simulink model "RLrobot"  (R2020b)
settings: Solver=ode15s  StartTime=0.0  StopTime=5  MaxStep=0.01  RelTol=1e-3  EnableMultiTasking=on
values from neighbouring files (symbols this model uses):
  Tf = 5    [ddpg_train_test.m]
  Ts = 0.2    [ddpg_train_test.m]
undefined symbols (not defined in the file or in its folder): Extr_Data_Mesh, sigbuilder_block, X, Y, Z
libraries: sm_lib x140, nesl_utility x29, simulink x13, rllib x1, walkingRobotUtils2 x1
(part 1 of 4)
settings Model: Creator=jihan  LastModifiedBy=zhug4
settings DataIOCC: LimitDataPoints=on  MaxDataPoints=10000
settings OptimizationCC: LifeSpan=inf
settings DebuggingCC: AllowSymbolicDim=off  SFUnexpectedBacktrackingDiag=warning  SFNoUnconditionalDefaultTransitionDiag=warning  SFExecutionAtInitializationDiag=none  ArithmeticOperatorsInVariantConditions=warning
settings SFSimCC: SimUseLocalCustomCode=off  CustomCodeUndefinedFunction=UseInterfaceOnly
settings RTWCC: RTWUseLocalCustomCode=off
settings CodeAppCC: StateflowObjectComments=on
settings GRTTargetCC: TargetLangStandard=C89/C90 (ANSI)
settings ConfigComp: CovMetricSettings=dw  CovSaveCumulativeToWorkspaceVar=on  CovSaveSingleToWorkspaceVar=on  CovExternalEMLEnable=off  CovSFcnEnable=off
settings SimscapeCC: SimscapeLogType=all  SimscapeLogSimulationStatistics=on  SimscapeLogDataHistory=10000

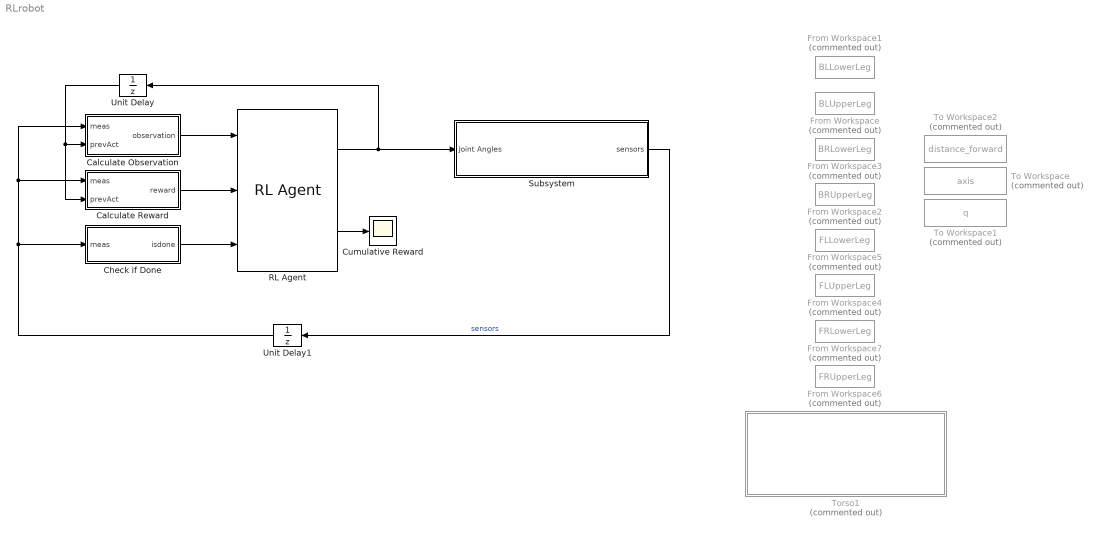
== system RLrobot ==
  Calculate Observation : Subsystem
  Calculate Reward : Subsystem
  Check if Done : Subsystem
  Cumulative Reward : Scope
  From Workspace : FromWorkspace  Commented=on  VariableName=BLUpperLeg
  From Workspace1 : FromWorkspace  Commented=on  VariableName=BLLowerLeg
  From Workspace2 : FromWorkspace  Commented=on  VariableName=BRUpperLeg
  From Workspace3 : FromWorkspace  Commented=on  VariableName=BRLowerLeg
  From Workspace4 : FromWorkspace  Commented=on  VariableName=FLUpperLeg
  From Workspace5 : FromWorkspace  Commented=on  VariableName=FLLowerLeg
  From Workspace6 : FromWorkspace  Commented=on  VariableName=FRUpperLeg
  From Workspace7 : FromWorkspace  Commented=on  VariableName=FRLowerLeg
  RL Agent : rllib/RL Agent  Agent=agent  ProvideReward=on  ProvideIsDone=on  ProvideCumRwd=on  TreatAsDirectFeedthrough=on  CollectLoggedSignals=on  CollectModelStates=on
      settings: SourceProductName=Reinforcement Learning
  Subsystem : Subsystem
  To Workspace : ToWorkspace  Commented=on  VariableName=axis  SaveFormat=Timeseries  SampleTime=1
      settings: MaxDataPoints=200
  To Workspace1 : ToWorkspace  Commented=on  VariableName=q  SaveFormat=Timeseries  SampleTime=1
      settings: MaxDataPoints=200
  To Workspace2 : ToWorkspace  Commented=on  VariableName=distance_forward  SaveFormat=Timeseries  SampleTime=1
      settings: MaxDataPoints=200
  Torso1 : Subsystem  Commented=on  mask{L=72, W=30, H=18, weight=20, rgb=[0 0.4 0.6], Lo=6, Lh=4}
      mask prompts: L "Length (cm)"; W "Width (cm)"; H "Thickness (cm)"; weight "Mass (kg)"; rgb "Color (rgb)"; Lo "Leg-Body Length offset"; Lh "Leg-Body Height offset"
      settings: PortSchema="{\"entries\":[{\"content\":{\"sides\":[{\"content\":{\"connectorIds\":[]},\"type\":\"ConnectorPlacement.EquallySpacedRectSide\",\"uuid\":\"a5f9388a-3463-4939-824e-c198da670e8b\"},{\"content\":{\"connectorIds\":[],\"side\":\"RIGHT\"},\"type\":\"ConnectorPlacement.EquallySpacedRectSide\",\"uuid\":\"721d6b97-2d6f-40dc-acf2-829076b6800c\"},{\"content\":{\"connectorIds\":[\"LConn1\",\"LConn2\"],\"side\":\"TOP\"},\"type\":\"ConnectorPlacement.EquallySpacedRectSide\",\"uuid\":\"81892bad-b270-4b55-8468-6b6312875fb4\"},{\"content\":{\"connectorIds\":[\"RConn1\",\"RConn2\",\"RConn3\",\"RConn4\"],\"side\":\"BOTTOM\"},\"type\":\"ConnectorPlacement.EquallySpacedRectSide\",\"uuid\":\"33367d70-bee6-41a0-95af-0235c6937548\"}]},\"type\":\"ConnectorPlacement.EquallySpacedConnector\",\"uuid\":\"7850cfb1-cafa-49f7-b14e-b890040a623d\"}],\"packageUris\":[\"http://schema.mathworks.com/mf0/Connector/R2020b\"],\"version\":\"1.0\"}"
  Unit Delay : UnitDelay  SampleTime=-1  HasFrameUpgradeWarning=on
  Unit Delay1 : UnitDelay  SampleTime=-1  HasFrameUpgradeWarning=on
  wires:
  Check if Done/1(isdone) -> RL Agent/3
  RL Agent/1 -> Subsystem/1(Joint Angles), Unit Delay/1
  Unit Delay/1 -> Calculate Reward/2(prevAct), Calculate Observation/2(prevAct)
  RL Agent/2 -> Cumulative Reward/1
  Calculate Observation/1(observation) -> RL Agent/1
  Calculate Reward/1(reward) -> RL Agent/2
  Subsystem/1(sensors) -> Unit Delay1/1  "sensors"
  Unit Delay1/1 -> Calculate Observation/1(meas), Calculate Reward/1(meas), Check if Done/1(meas)

== system RLrobot/Calculate Observation ==
  meas : Inport
  prevAct : Inport  Port=2
  Bus Selector : BusSelector  OutputSignals=yaw,pitch,roll,wx,wy,wz,bx,by,bz,x,y,z,vx,vy,vz,ax,ay,az
  Mux : Mux  Inputs=19
  Rate Transition : RateTransition
  Scale Height : Gain  Gain=1/0.05
  Subtract Initial Height : Bias
  observation : Outport  VectorParamsAs1DForOutWhenUnconnected=off
  wires:
  meas/1 -> Bus Selector/1
  Mux/1 -> Rate Transition/1
  Rate Transition/1 -> observation/1
  Subtract Initial Height/1 -> Scale Height/1
  prevAct/1 -> Mux/19
  Bus Selector/1 -> Mux/1  "<yaw>"
  Bus Selector/2 -> Mux/2  "<pitch>"
  Bus Selector/3 -> Mux/3  "<roll>"
  Bus Selector/4 -> Mux/4  "<wx>"
  Bus Selector/5 -> Mux/5  "<wy>"
  Bus Selector/6 -> Mux/6  "<wz>"
  Bus Selector/7 -> Mux/7  "<bx>"
  Bus Selector/8 -> Mux/8  "<by>"
  Bus Selector/9 -> Mux/9  "<bz>"
  Bus Selector/10 -> Mux/10  "<x>"
  Bus Selector/11 -> Mux/11  "<y>"
  Bus Selector/12 -> Subtract Initial Height/1  "<z>"
  Scale Height/1 -> Mux/12  "Z_scaled"
  Bus Selector/13 -> Mux/13  "<vx>"
  Bus Selector/14 -> Mux/14  "<vy>"
  Bus Selector/15 -> Mux/15  "<vz>"
  Bus Selector/16 -> Mux/16  "<ax>"
  Bus Selector/17 -> Mux/17  "<ay>"
  Bus Selector/18 -> Mux/18  "<az>"

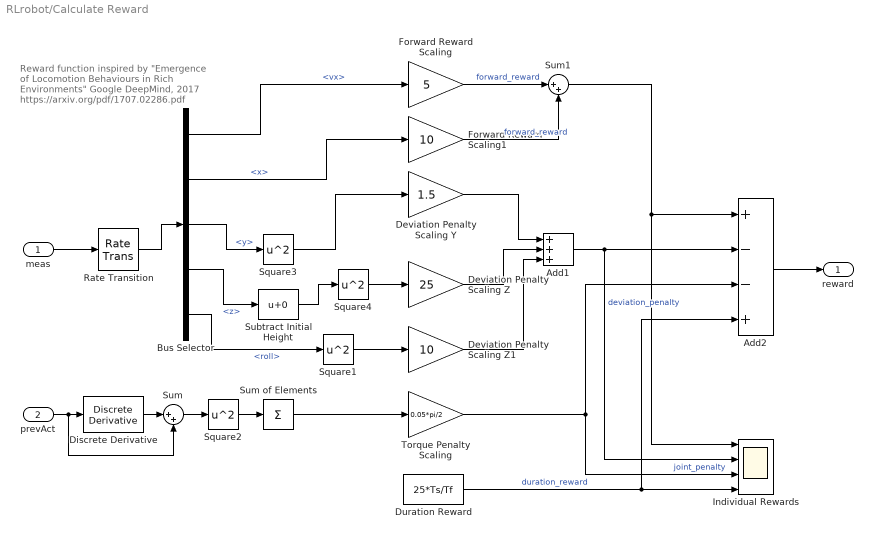
== system RLrobot/Calculate Reward ==
  note: Reward function inspired by
      | "Emergence of Locomotion Behaviours in Rich Environments"
      | Google DeepMind, 2017
      | https://arxiv.org/pdf/1707.02286.pdf
  meas : Inport
  prevAct : Inport  Port=2
  Add1 : Sum  Inputs=+++
  Add2 : Sum  Inputs=+--+
  Bus Selector : BusSelector  OutputSignals=vx,x,y,z,roll
  Deviation Penalty Scaling Y : Gain  Gain=1.5
  Deviation Penalty Scaling Z : Gain  Gain=25
  Deviation Penalty Scaling Z1 : Gain  Gain=10
  Discrete Derivative : simulink/Discrete/Discrete Derivative  gainval=1.0  ICPrevScaledInput=0.0  OutMin=[]  OutMax=[]  OutDataType=fixdt(1, 16)  OutScaling=2^-10  DoSatur=off
  Duration Reward : Constant  Value=25*Ts/Tf
  Forward Reward Scaling : Gain  Gain=5
  Forward Reward Scaling1 : Gain  Gain=10
  Individual Rewards : Scope  NumInputPorts=4
  Rate Transition : RateTransition  OutPortSampleTime=Ts
  Square{1..4} (4 alike) : Math  Operator=square  SignedPower=on  SaturateOnIntegerOverflow=on
  Subtract Initial Height : Bias
  Sum : Sum  Inputs=|++
  Sum of Elements : Sum  Inputs=+
  Sum1 : Sum  Inputs=|++
  Torque Penalty Scaling : Gain  Gain=0.05*pi/2
  reward : Outport  VectorParamsAs1DForOutWhenUnconnected=off
  wires:
  Add2/1 -> reward/1
  Add1/1 -> Add2/2, Individual Rewards/2  "deviation_penalty"
  Sum of Elements/1 -> Torque Penalty Scaling/1
  Bus Selector/1 -> Forward Reward Scaling/1  "<vx>"
  Square3/1 -> Deviation Penalty Scaling Y/1
  Duration Reward/1 -> Individual Rewards/4, Add2/4  "duration_reward"
  Square2/1 -> Sum of Elements/1
  Torque Penalty Scaling/1 -> Add2/3, Individual Rewards/3  "joint_penalty"
  Square4/1 -> Deviation Penalty Scaling Z/1
  Subtract Initial Height/1 -> Square4/1
  Deviation Penalty Scaling Z/1 -> Add1/2
  Deviation Penalty Scaling Y/1 -> Add1/1
  Bus Selector/3 -> Square3/1  "<y>"
  Bus Selector/4 -> Subtract Initial Height/1  "<z>"
  Rate Transition/1 -> Bus Selector/1
  meas/1 -> Rate Transition/1
  prevAct/1 -> Sum/2, Discrete Derivative/1
  Discrete Derivative/1 -> Sum/1
  Sum/1 -> Square2/1
  Bus Selector/2 -> Forward Reward Scaling1/1  "<x>"
  Sum1/1 -> Add2/1, Individual Rewards/1
  Forward Reward Scaling/1 -> Sum1/1  "forward_reward"
  Forward Reward Scaling1/1 -> Sum1/2  "forward_reward"
  Deviation Penalty Scaling Z1/1 -> Add1/3
  Bus Selector/5 -> Square1/1  "<roll>"
  Square1/1 -> Deviation Penalty Scaling Z1/1

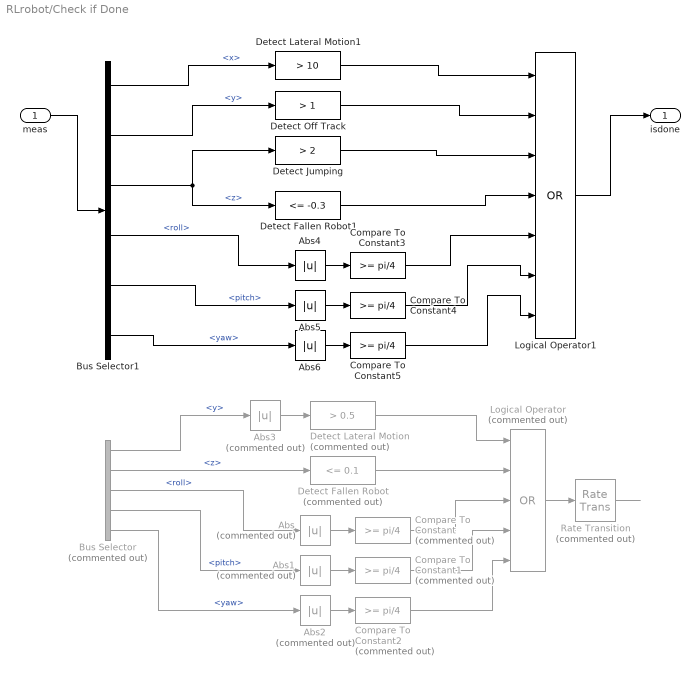
== system RLrobot/Check if Done ==
  meas : Inport
  Abs{,1..3} (4 alike) : Abs  Commented=on
  Abs4 : Abs
  Abs5 : Abs
  Abs6 : Abs
  Bus Selector : BusSelector  Commented=on  OutputSignals=y,z,roll,pitch,yaw
  Bus Selector1 : BusSelector  OutputSignals=x,y,z,roll,pitch,yaw
  Compare To Constant : simulink/Logic and Bit Operations/Compare To Constant  Commented=on  relop=>=  const=pi/4  OutDataTypeStr=boolean
  Compare To Constant1 : simulink/Logic and Bit Operations/Compare To Constant  Commented=on  relop=>=  const=pi/4  OutDataTypeStr=boolean
  Compare To Constant2 : simulink/Logic and Bit Operations/Compare To Constant  Commented=on  relop=>=  const=pi/4  OutDataTypeStr=boolean
  Compare To Constant3 : simulink/Logic and Bit Operations/Compare To Constant  relop=>=  const=pi/4  OutDataTypeStr=boolean
  Compare To Constant4 : simulink/Logic and Bit Operations/Compare To Constant  relop=>=  const=pi/4  OutDataTypeStr=boolean
  Compare To Constant5 : simulink/Logic and Bit Operations/Compare To Constant  relop=>=  const=pi/4  OutDataTypeStr=boolean
  Detect Fallen Robot : simulink/Logic and Bit Operations/Compare To Constant  Commented=on  relop=<=  const=0.1  OutDataTypeStr=boolean
  Detect Fallen Robot1 : simulink/Logic and Bit Operations/Compare To Constant  relop=<=  const=-0.3  OutDataTypeStr=boolean
  Detect Jumping : simulink/Logic and Bit Operations/Compare To Constant  relop=>  const=2  OutDataTypeStr=boolean
  Detect Lateral Motion : simulink/Logic and Bit Operations/Compare To Constant  Commented=on  relop=>  const=0.5  OutDataTypeStr=boolean
  Detect Lateral Motion1 : simulink/Logic and Bit Operations/Compare To Constant  relop=>  const=10  OutDataTypeStr=boolean
  Detect Off Track : simulink/Logic and Bit Operations/Compare To Constant  relop=>  const=1  OutDataTypeStr=boolean
  Logical Operator : Logic  Commented=on  Operator=OR  Inputs=5  AllPortsSameDT=off  OutDataTypeStr=boolean
  Logical Operator1 : Logic  Operator=OR  Inputs=7  AllPortsSameDT=off  OutDataTypeStr=boolean
  Rate Transition : RateTransition  Commented=on
  isdone : Outport  VectorParamsAs1DForOutWhenUnconnected=off
  wires:
  Bus Selector/5 -> Abs2/1  "<yaw>"
  Abs2/1 -> Compare To Constant2/1
  Abs3/1 -> Detect Lateral Motion/1
  Detect Lateral Motion/1 -> Logical Operator/1
  Bus Selector/3 -> Abs/1  "<roll>"
  Abs1/1 -> Compare To Constant1/1
  Abs/1 -> Compare To Constant/1
  Compare To Constant2/1 -> Logical Operator/5
  Logical Operator/1 -> Rate Transition/1
  Compare To Constant/1 -> Logical Operator/3
  Compare To Constant1/1 -> Logical Operator/4
  Bus Selector/1 -> Abs3/1  "<y>"
  Bus Selector/4 -> Abs1/1  "<pitch>"
  Detect Fallen Robot/1 -> Logical Operator/2
  Bus Selector/2 -> Detect Fallen Robot/1  "<z>"
  Rate Transition/1 -> ?
  meas/1 -> Bus Selector1/1
  Bus Selector1/1 -> Detect Lateral Motion1/1  "<x>"
  Detect Lateral Motion1/1 -> Logical Operator1/1
  Logical Operator1/1 -> isdone/1
  Detect Fallen Robot1/1 -> Logical Operator1/4
  Bus Selector1/2 -> Detect Off Track/1  "<y>"
  Detect Off Track/1 -> Logical Operator1/2
  Detect Jumping/1 -> Logical Operator1/3
  Bus Selector1/3 -> Detect Fallen Robot1/1, Detect Jumping/1  "<z>"
  Abs4/1 -> Compare To Constant3/1
  Compare To Constant5/1 -> Logical Operator1/7
  Compare To Constant4/1 -> Logical Operator1/6
  Abs6/1 -> Compare To Constant5/1
  Abs5/1 -> Compare To Constant4/1
  Bus Selector1/4 -> Abs4/1  "<roll>"
  Bus Selector1/5 -> Abs5/1  "<pitch>"
  Compare To Constant3/1 -> Logical Operator1/5
  Bus Selector1/6 -> Abs6/1  "<yaw>"

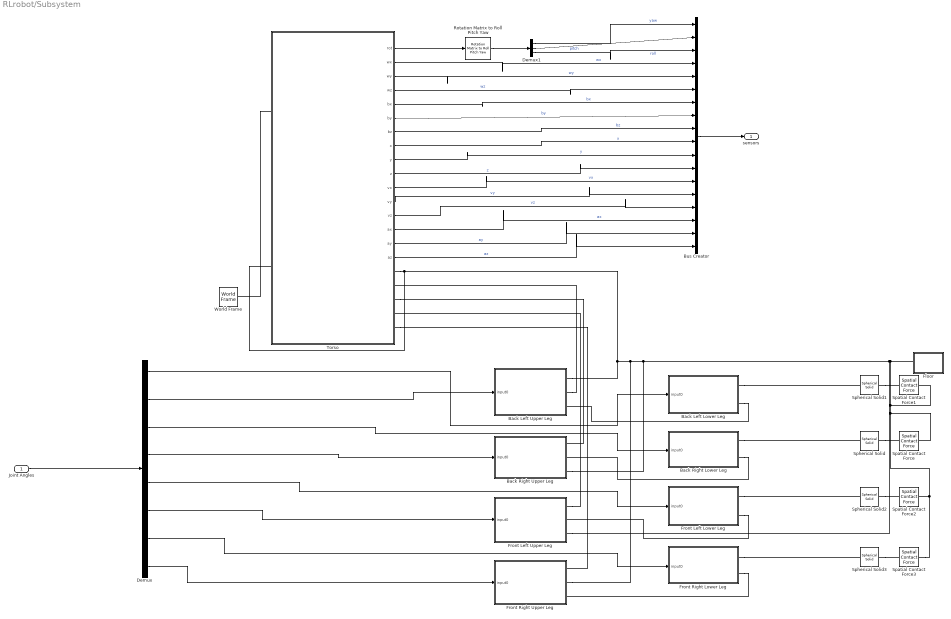
== system RLrobot/Subsystem ==
  Joint Angles : Inport  Unit=m^2*kg/s^2
  " Front Right Upper Leg" : Subsystem  mask{L=7, W=5, H=25, weight=1, rgb=[0 0.4 0.6]}
      mask prompts: L "Length (cm)"; W "Width (cm)"; H "Height (cm)"; weight "Weight (kg)"; rgb "Color (rgb)"
  Back Left Lower Leg : Subsystem  mask{L=7, W=5, H=25, weight=1, rgb=[0 0.4 0.6]}
      mask prompts: L "Length (cm)"; W "Width (cm)"; H "Height (cm)"; weight "Weight (cm)"; rgb "Color (rgb)"
  Back Left Upper Leg : Subsystem  mask{L=7, W=5, H=25, weight=1, rgb=[0 0.4 0.6]}
      mask prompts: L "Length (cm)"; W "Width (cm)"; H "Height (cm)"; weight "Weight (cm)"; rgb "Color (rgb)"
  Back Right Lower Leg : Subsystem  mask{L=7, W=5, H=25, weight=1, rgb=[0 0.4 0.6]}
      mask prompts: L "Length (cm)"; W "Width (cm)"; H "Height (cm)"; weight "Weight (cm)"; rgb "Color (rgb)"
  Back Right Upper Leg : Subsystem  mask{L=7, W=5, H=25, weight=1, rgb=[0 0.4 0.6]}
      mask prompts: L "Length (cm)"; W "Width (cm)"; H "Height (cm)"; weight "Weight (kg)"; rgb "Color (rgb)"
  Bus Creator : BusCreator  Inputs=18
  Demux : Demux  Outputs=8
  Demux1 : Demux  Outputs=3
  Floor : Subsystem  mask{xyz=[0 1 0], floor_angle=0, offset=90}
      mask prompts: xyz "Axis of Rotation [x y z]"; floor_angle "Angle of Rotation (deg)"; offset "Floor Offset (cm)"
      settings: PortSchema="{\"entries\":[{\"content\":{\"sides\":[{\"content\":{\"connectorIds\":[]},\"type\":\"ConnectorPlacement.EquallySpacedRectSide\",\"uuid\":\"11e96fa0-1698-473b-91b9-c65afd80511d\"},{\"content\":{\"connectorIds\":[],\"side\":\"RIGHT\"},\"type\":\"ConnectorPlacement.EquallySpacedRectSide\",\"uuid\":\"698adcb8-63bc-493a-8506-9415d482b8fe\"},{\"content\":{\"connectorIds\":[\"LConn1\"],\"side\":\"TOP\"},\"type\":\"ConnectorPlacement.EquallySpacedRectSide\",\"uuid\":\"168764b1-d6dd-4696-94dd-d7ccb4fea120\"}]},\"type\":\"ConnectorPlacement.EquallySpacedConnector\",\"uuid\":\"ee92c37f-2eb0-4cad-ab84-9513ea85ac02\"}],\"packageUris\":[\"http://schema.mathworks.com/mf0/Connector/19700101\"],\"version\":\"1.0\"}"
  Front Left Lower Leg : Subsystem  mask{L=7, W=5, H=25, weight=1, rgb=[0 0.4 0.6]}
      mask prompts: L "Length (cm)"; W "Width (cm)"; H "Height (cm)"; weight "Weight (kg)"; rgb "Color (rgb)"
  Front Left Upper Leg : Subsystem  mask{L=7, W=5, H=25, weight=1, rgb=[0 0.4 0.6]}
      mask prompts: L "Length (cm)"; W "Width (cm)"; H "Height (cm)"; weight "Weight (kg)"; rgb "Color (rgb)"
  Front Right Lower Leg : Subsystem  mask{L=7, W=5, H=25, weight=1, rgb=[0 0.4 0.6]}
      mask prompts: L "Length (cm)"; W "Width (cm)"; H "Height (cm)"; weight "Weight (cm)"; rgb "Color (rgb)"
  Rotation Matrix to Roll Pitch Yaw : walkingRobotUtils2/Rotation Matrix to  Roll Pitch Yaw  SystemSampleTime=-1  VariantActivationTime=update diagram  Latency=0  AutoFrameSizeCalculation=off
  Spatial Contact Force{,1..3} (4 alike) : sm_lib/Forces and Torques/Spatial Contact Force  CoefficientOfDynamicFriction=0.3  CoefficientOfStaticFriction=0.3  NormalDamping=1e3  NormalDampingUnits=N/(m/s)  NormalStiffness=1e6  NormalStiffnessUnits=N/m  FrictionalCriticalVelocity=1e-3  FrictionalCriticalVelocityUnits=m/s  ZeroCrossDetectContactStartAndEnd=off  SenseFrictionalForceMagnitude=off  SenseNormalForceMagnitude=off  SenseSeparationDistance=off  NormalTransitionRegionWidth=1e-4  NormalTransitionRegionWidthUnits=m  FrictionType=SmoothStickSlip
  Spherical Solid{,1..3} (4 alike) : sm_lib/Body Elements/Spherical Solid  GraphicAmbientColor=[0.15 0.15 0.15 1.0]  BasedOnType=Density  CenterOfMass=[0 0 0]  CenterOfMassUnits=m  GraphicDiffuseColor=[0.5 0.5 0.5]  Density=1000  DensityUnits=kg/m^3  DoExposeReferenceFrame=on  GraphicEmissiveColor=[0.0 0.0 0.0 1.0]  ExportEntireGeometry=on  SerializedExposedGeometries=<ExposedGeometries><ExposedGeometry><RawGeometryId>entire</RawGeometryId><ExposedGeometryId>G</ExposedGeometryId></ExposedGeometry></ExposedGeometries>  SerializedFrames=<Frames/>  MarkerShape=Sphere  MarkerSize=10  GraphicType=FromGeometry  InertiaType=CalculateFromGeometry  Mass=1  MassUnits=kg  MomentsOfInertia=[1 1 1]  MomentsOfInertiaUnits=kg*m^2  GraphicOpacity=1.0  ProductsOfInertia=[0 0 0]  ProductsOfInertiaUnits=kg*m^2  GraphicShininess=75  GraphicSpecularColor=[0.5 0.5 0.5 1.0]  SphereRadius=4  SphereRadiusUnits=cm  GraphicVisPropType=SimpleVisualProperties
  Torso : Subsystem  mask{L=72, W=30, H=18, weight=20, rgb=[0 0.4 0.6], Lo=6, Lh=4}
      mask prompts: L "Length (cm)"; W "Width (cm)"; H "Thickness (cm)"; weight "Mass (kg)"; rgb "Color (rgb)"; Lo "Leg-Body Length offset"; Lh "Leg-Body Height offset"
  World Frame : sm_lib/Frames and Transforms/World Frame
  sensors : Outport
  wires:
  Demux/1 -> Back Left Lower Leg/1(input0)
  Demux/3 -> Back Right Lower Leg/1(input0)
  Demux/5 -> Front Left Lower Leg/1(input0)
  Demux/4 -> Back Right Upper Leg/1(input0)
  Demux/8 -> " Front Right Upper Leg"/1(input0)
  Demux/6 -> Front Left Upper Leg/1(input0)
  Demux/7 -> Front Right Lower Leg/1(input0)
  Demux/2 -> Back Left Upper Leg/1(input0)
  Joint Angles/1 -> Demux/1
  Bus Creator/1 -> sensors/1
  Demux1/3 -> Bus Creator/3  "roll"
  Demux1/1 -> Bus Creator/1  "yaw"
  Demux1/2 -> Bus Creator/2  "pitch"
  Torso/2(wx) -> Bus Creator/4  "wx"
  Torso/3(wy) -> Bus Creator/5  "wy"
  Torso/4(wz) -> Bus Creator/6  "wz"
  Torso/5(bx) -> Bus Creator/7  "bx"
  Torso/6(by) -> Bus Creator/8  "by"
  Torso/7(bz) -> Bus Creator/9  "bz"
  Torso/8(x) -> Bus Creator/10  "x"
  Torso/9(y) -> Bus Creator/11  "y"
  Torso/10(z) -> Bus Creator/12  "z"
  Torso/11(vx) -> Bus Creator/13  "vx"
  Torso/12(vy) -> Bus Creator/14  "vy"
  Torso/13(vz) -> Bus Creator/15  "vz"
  Torso/15(ay) -> Bus Creator/17  "ay"
  Torso/14(ax) -> Bus Creator/16  "ax"
  Torso/16(az) -> Bus Creator/18  "az"
  Torso/1(rot) -> Rotation Matrix to Roll Pitch Yaw/1
  Rotation Matrix to Roll Pitch Yaw/1 -> Demux1/1
  connections:
  Back Left Lower Leg/RConn2 -- Back Left Upper Leg/RConn3
  Spatial Contact Force1/RConn1 -- Spatial Contact Force3/RConn1 -- Spatial Contact Force2/RConn1 -- Spatial Contact Force/RConn1 -- Floor/LConn1 -- Torso/RConn1 -- Torso/LConn2 -- Back Left Upper Leg/RConn1 -- " Front Right Upper Leg"/RConn2 -- Back Right Upper Leg/RConn3 -- Front Left Upper Leg/RConn3
  Spherical Solid3/LConn1 -- Spatial Contact Force3/LConn1
  Spherical Solid/LConn1 -- Spatial Contact Force/LConn1
  Back Right Lower Leg/RConn1 -- Spherical Solid/RConn1
  Spherical Solid1/LConn1 -- Spatial Contact Force1/LConn1
  Front Left Lower Leg/RConn1 -- Spherical Solid2/RConn1
  Back Left Upper Leg/RConn2 -- Torso/RConn2
  Spherical Solid2/LConn1 -- Spatial Contact Force2/LConn1
  Front Right Lower Leg/RConn2 -- " Front Right Upper Leg"/RConn3
  Back Right Lower Leg/RConn2 -- Back Right Upper Leg/RConn2
  Back Left Lower Leg/RConn1 -- Spherical Solid1/RConn1
  Front Right Lower Leg/RConn1 -- Spherical Solid3/RConn1
  Torso/RConn5 -- " Front Right Upper Leg"/RConn1
  Front Left Lower Leg/RConn2 -- Front Left Upper Leg/RConn2
  Torso/LConn1 -- World Frame/RConn1
  Front Left Upper Leg/RConn1 -- Torso/RConn4
  Torso/RConn3 -- Back Right Upper Leg/RConn1

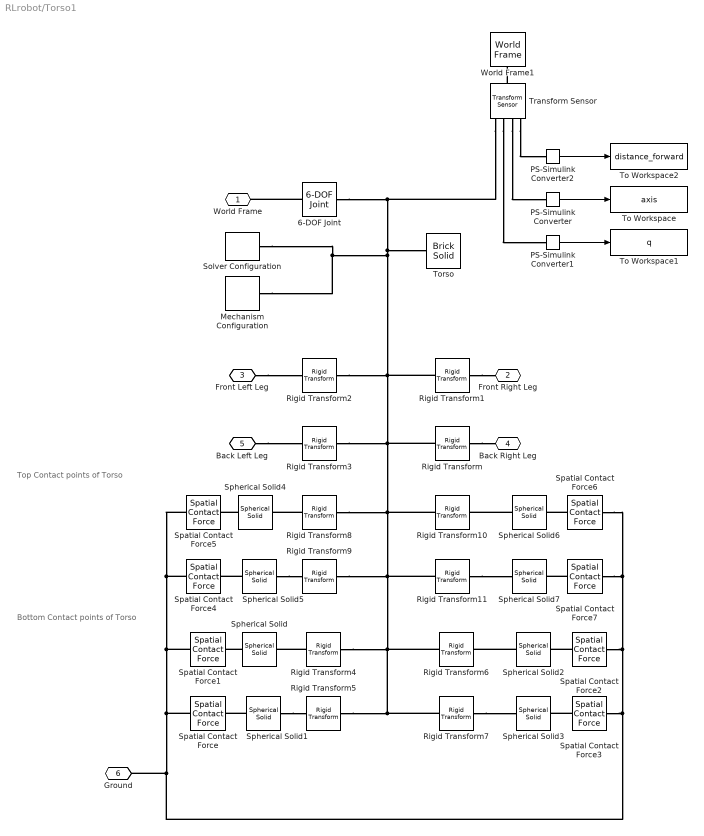
== system RLrobot/Torso1 ==
  note: Top Contact points of Torso
  note: Bottom Contact points of Torso
  6-DOF Joint : sm_lib/Joints/6-DOF Joint  JointMode=Normal  SenseConstraintForce=off  SenseConstraintForceX=off  SenseConstraintForceY=off  SenseConstraintForceZ=off  SenseConstraintTorque=off  SenseConstraintTorqueX=off  SenseConstraintTorqueY=off  SenseConstraintTorqueZ=off  SenseTotalForce=off  SenseTotalForceX=off  SenseTotalForceY=off  SenseTotalForceZ=off  SenseTotalTorque=off  SenseTotalTorqueX=off  SenseTotalTorqueY=off  SenseTotalTorqueZ=off  CompositeWrenchDir=FollowerOnBase  CompositeWrenchFrame=BaseFrame  PxEquilibriumPosition=0  PxEquilibriumPositionUnits=m  PxSpringStiffness=0  PxSpringStiffnessUnits=N/m  PxDampingCoefficient=0  PxDampingCoefficientUnits=N/(m/s)  PxTorqueActuationMode=NoTorque  PxMotionActuationMode=ComputedMotion  PxSensePosition=off  PxSenseVelocity=off  PxSenseAcceleration=off  PxSenseTorqueForce=off  PxSenseLowerLimitTorqueForce=off  PxSenseUpperLimitTorqueForce=off  PxLowerLimitSpecify=off  PxLowerLimitBound=-1  PxLowerLimitBoundUnits=m  PxLowerLimitStiffness=1e6  PxLowerLimitStiffnessUnits=N/m  PxLowerLimitDamping=1e3  PxLowerLimitDampingUnits=N/(m/s)  PxLowerLimitTransitionRegionWidth=1e-4  PxLowerLimitTransitionRegionWidthUnits=m  PxUpperLimitSpecify=off  PxUpperLimitBound=1  PxUpperLimitBoundUnits=m  PxUpperLimitStiffness=1e6  PxUpperLimitStiffnessUnits=N/m  PxUpperLimitDamping=1e3  PxUpperLimitDampingUnits=N/(m/s)  PxUpperLimitTransitionRegionWidth=1e-4  PxUpperLimitTransitionRegionWidthUnits=m  PxPositionTargetSpecify=off  PxPositionTargetPriority=High  PxPositionTargetValue=0  PxPositionTargetValueUnits=m  PxVelocityTargetSpecify=off  PxVelocityTargetPriority=High  PxVelocityTargetValue=0  PxVelocityTargetValueUnits=m/s  PyEquilibriumPosition=0  PyEquilibriumPositionUnits=m  PySpringStiffness=0  PySpringStiffnessUnits=N/m  PyDampingCoefficient=0  PyDampingCoefficientUnits=N/(m/s)  PyTorqueActuationMode=NoTorque  PyMotionActuationMode=ComputedMotion  PySensePosition=off  PySenseVelocity=off  PySenseAcceleration=off  PySenseTorqueForce=off  PySenseLowerLimitTorqueForce=off  PySenseUpperLimitTorqueForce=off  PyLowerLimitSpecify=off  PyLowerLimitBound=-1  PyLowerLimitBoundUnits=m  PyLowerLimitStiffness=1e6  PyLowerLimitStiffnessUnits=N/m  PyLowerLimitDamping=1e3  PyLowerLimitDampingUnits=N/(m/s)  PyLowerLimitTransitionRegionWidth=1e-4  PyLowerLimitTransitionRegionWidthUnits=m  PyUpperLimitSpecify=off  PyUpperLimitBound=1  PyUpperLimitBoundUnits=m  PyUpperLimitStiffness=1e6  PyUpperLimitStiffnessUnits=N/m  PyUpperLimitDamping=1e3  PyUpperLimitDampingUnits=N/(m/s)  PyUpperLimitTransitionRegionWidth=1e-4  PyUpperLimitTransitionRegionWidthUnits=m  PyPositionTargetSpecify=off  PyPositionTargetPriority=High  PyPositionTargetValue=0  PyPositionTargetValueUnits=m  PyVelocityTargetSpecify=off  PyVelocityTargetPriority=High  PyVelocityTargetValue=0  PyVelocityTargetValueUnits=m/s  PzEquilibriumPosition=0  PzEquilibriumPositionUnits=m  PzSpringStiffness=0  PzSpringStiffnessUnits=N/m  PzDampingCoefficient=0  PzDampingCoefficientUnits=N/(m/s)  PzTorqueActuationMode=NoTorque  PzMotionActuationMode=ComputedMotion  PzSensePosition=off  PzSenseVelocity=off  PzSenseAcceleration=off  PzSenseTorqueForce=off  PzSenseLowerLimitTorqueForce=off  PzSenseUpperLimitTorqueForce=off  PzLowerLimitSpecify=off  PzLowerLimitBound=-1  PzLowerLimitBoundUnits=m  PzLowerLimitStiffness=1e6  PzLowerLimitStiffnessUnits=N/m  PzLowerLimitDamping=1e3  PzLowerLimitDampingUnits=N/(m/s)  PzLowerLimitTransitionRegionWidth=1e-4  PzLowerLimitTransitionRegionWidthUnits=m  PzUpperLimitSpecify=off  PzUpperLimitBound=1  PzUpperLimitBoundUnits=m  PzUpperLimitStiffness=1e6  PzUpperLimitStiffnessUnits=N/m  PzUpperLimitDamping=1e3  PzUpperLimitDampingUnits=N/(m/s)  PzUpperLimitTransitionRegionWidth=1e-4  PzUpperLimitTransitionRegionWidthUnits=m  PzPositionTargetSpecify=off  PzPositionTargetPriority=High  PzPositionTargetValue=0  PzPositionTargetValueUnits=m  PzVelocityTargetSpecify=off  PzVelocityTargetPriority=High  PzVelocityTargetValue=0  PzVelocityTargetValueUnits=m/s  SphDefPosRotationMethod=None  SphDefPosRotationAngleUnits=deg  SphDefPosRotationStandardAxis=+Z  SphDefPosRotationAngle=0.0  SphDefPosRotationArbitraryAxis=[0 0 1]  SphDefPosFollAlignAxisA=+X  SphDefPosBaseAlignAxisA=+Y  SphDefPosFollAlignAxisB=+Y  SphDefPosBaseAlignAxisB=+Z  SphDefPosRotationSequenceAxes=FollowerAxes  SphDefPosRotationSequence=XYX  SphDefPosRotationSequenceAngles=[0 0 0]  SphDefPosRotationSequenceAnglesUnits=deg  SphDefPosRotationMatrix=[1 0 0; 0 1 0; 0 0 1]  SphEqPosRotationMethod=None  SphEqPosRotationAngleUnits=deg  SphEqPosRotationStandardAxis=+Z  SphEqPosRotationAngle=0.0  SphEqPosRotationArbitraryAxis=[0 0 1]  SphEqPosFollAlignAxisA=+X  SphEqPosBaseAlignAxisA=+Y  SphEqPosFollAlignAxisB=+Y  SphEqPosBaseAlignAxisB=+Z  SphEqPosRotationSequenceAxes=FollowerAxes  SphEqPosRotationSequence=XYX  SphEqPosRotationSequenceAngles=[0 0 0]  SphEqPosRotationSequenceAnglesUnits=deg  SphEqPosRotationMatrix=[1 0 0; 0 1 0; 0 0 1]  SphSpringStiffness=0  SphSpringStiffnessUnits=N*m/deg  SphDampingCoefficient=0  SphDampingCoefficientUnits=N*m/(deg/s)  SphActuateTorqueX=off  SphActuateTorqueY=off  SphActuateTorqueZ=off  SphActuateTorque=off  SphTorqueActuationMode=NoTorque  SphMotionActuationMode=ComputedMotion  SphActuationFrame=BaseFrame  SphSensePosition=off  SphSenseVelocityX=off  SphSenseVelocityY=off  SphSenseVelocityZ=off  SphSenseVelocity=off  SphSenseAccelerationX=off  SphSenseAccelerationY=off  SphSenseAccelerationZ=off  SphSenseAcceleration=off  SphSenseTorqueX=off  SphSenseTorqueY=off  SphSenseTorqueZ=off  SphSenseTorqueForce=off  SphSenseLowerLimitTorqueMag=off  SphSenseUpperLimitTorqueMag=off  SphSensingFrame=BaseFrame  SphLowerLimitSpecify=off  SphLowerLimitBound=15  SphLowerLimitBoundUnits=deg  SphLowerLimitStiffness=1e4  SphLowerLimitStiffnessUnits=N*m/deg  SphLowerLimitDamping=10  SphLowerLimitDampingUnits=N*m/(deg/s)  SphLowerLimitTransitionRegionWidth=0.1  SphLowerLimitTransitionRegionWidthUnits=deg  SphUpperLimitSpecify=off  SphUpperLimitBound=45  SphUpperLimitBoundUnits=deg  SphUpperLimitStiffness=1e4  SphUpperLimitStiffnessUnits=N*m/deg  SphUpperLimitDamping=10  SphUpperLimitDampingUnits=N*m/(deg/s)  SphUpperLimitTransitionRegionWidth=0.1  SphUpperLimitTransitionRegionWidthUnits=deg  SphPositionTargetRotationMethod=None  SphPositionTargetRotationAngleUnits=deg  SphPositionTargetRotationStandardAxis=+Z  SphPositionTargetRotationAngle=0.0  SphPositionTargetRotationArbitraryAxis=[0 0 1]  SphPositionTargetFollAlignAxisA=+X  SphPositionTargetBaseAlignAxisA=+Y  SphPositionTargetFollAlignAxisB=+Y  SphPositionTargetBaseAlignAxisB=+Z  SphPositionTargetRotationSequenceAxes=FollowerAxes  SphPositionTargetRotationSequence=XYX  SphPositionTargetRotationSequenceAngles=[0 0 0]  SphPositionTargetRotationSequenceAnglesUnits=deg  SphPositionTargetRotationMatrix=[1 0 0; 0 1 0; 0 0 1]  SphPositionTargetSpecify=off  SphPositionTargetPriority=High  SphVelocityTargetValue=[0 0 0]  SphVelocityTargetValueUnits=deg/s  SphVelocityTargetSpecify=off  SphVelocityTargetPriority=High  SphVelocityTargetInFollowerFrame=on
  Mechanism Configuration : sm_lib/Utilities/Mechanism Configuration  UniformGravity=Constant  GravityVector=[0 0 -9.80665]  GravityVectorUnits=m/s^2  GravityUnits=m/s^2  LinearizationDelta=0.001  JointModeTransitionNonlinearIterations=2
  PS-Simulink Converter : nesl_utility/PS-Simulink Converter  PhysicalDomain=network_engine_domain  SubClassName=ps_output  LeftPortType=input  RightPortType=output  PseudoPeriodic=off  Frequencies=[]  Unit=inherit  AffineConversion=off
  PS-Simulink Converter1 : nesl_utility/PS-Simulink Converter  PhysicalDomain=network_engine_domain  SubClassName=ps_output  LeftPortType=input  RightPortType=output  PseudoPeriodic=off  Frequencies=[]  Unit=inherit  AffineConversion=off
  PS-Simulink Converter2 : nesl_utility/PS-Simulink Converter  PhysicalDomain=network_engine_domain  SubClassName=ps_output  LeftPortType=input  RightPortType=output  PseudoPeriodic=off  Frequencies=[]  Unit=inherit  AffineConversion=off
  Rigid Transform : sm_lib/Frames and Transforms/Rigid Transform  TranslationMethod=Cartesian  TranslationStandardOffset=L/2  TranslationLengthUnit=cm  TranslationStandardAxis=+X  TranslationCartesianOffset=[-L/2+Lo W/2 -H/2+Lh]  TranslationROffset=0  TranslationROffsetUnits=m  TranslationZOffset=0  TranslationZOffsetUnits=m  TranslationThetaOffset=0  TranslationThetaOffsetUnits=deg  RotationMethod=StandardAxis  RotationAngleUnits=deg  RotationStandardAxis=-X  RotationAngle=90  RotationArbitraryAxis=[0 0 1]  FollAlignAxisA=+X  BaseAlignAxisA=+Y  FollAlignAxisB=+Y  BaseAlignAxisB=+Z  RotationSequenceAxes=FollowerAxes  RotationSequence=XYX  RotationSequenceAngles=[0 0 0]  RotationSequenceAnglesUnits=deg  RotationMatrix=[1 0 0; 0 1 0; 0 0 1]
  Rigid Transform1 : sm_lib/Frames and Transforms/Rigid Transform  TranslationMethod=Cartesian  TranslationStandardOffset=L/2  TranslationLengthUnit=cm  TranslationStandardAxis=-X  TranslationCartesianOffset=[L/2-Lo W/2 -H/2+Lh]  TranslationROffset=0  TranslationROffsetUnits=m  TranslationZOffset=0  TranslationZOffsetUnits=m  TranslationThetaOffset=0  TranslationThetaOffsetUnits=deg  RotationMethod=StandardAxis  RotationAngleUnits=deg  RotationStandardAxis=-X  RotationAngle=90  RotationArbitraryAxis=[0 0 1]  FollAlignAxisA=+X  BaseAlignAxisA=+Y  FollAlignAxisB=+Y  BaseAlignAxisB=+Z  RotationSequenceAxes=FollowerAxes  RotationSequence=XYX  RotationSequenceAngles=[0 0 0]  RotationSequenceAnglesUnits=deg  RotationMatrix=[1 0 0; 0 1 0; 0 0 1]
  Rigid Transform10 : sm_lib/Frames and Transforms/Rigid Transform  TranslationMethod=Cartesian  TranslationStandardOffset=L/2  TranslationLengthUnit=cm  TranslationStandardAxis=-X  TranslationCartesianOffset=[L/2 W/2 H/2]  TranslationROffset=0  TranslationROffsetUnits=m  TranslationZOffset=0  TranslationZOffsetUnits=m  TranslationThetaOffset=0  TranslationThetaOffsetUnits=deg  RotationMethod=StandardAxis  RotationAngleUnits=deg  RotationStandardAxis=-X  RotationAngle=90  RotationArbitraryAxis=[0 0 1]  FollAlignAxisA=+X  BaseAlignAxisA=+Y  FollAlignAxisB=+Y  BaseAlignAxisB=+Z  RotationSequenceAxes=FollowerAxes  RotationSequence=XYX  RotationSequenceAngles=[0 0 0]  RotationSequenceAnglesUnits=deg  RotationMatrix=[1 0 0; 0 1 0; 0 0 1]
  Rigid Transform11 : sm_lib/Frames and Transforms/Rigid Transform  TranslationMethod=Cartesian  TranslationStandardOffset=L/2  TranslationLengthUnit=cm  TranslationStandardAxis=+X  TranslationCartesianOffset=[-L/2 W/2 H/2]  TranslationROffset=0  TranslationROffsetUnits=m  TranslationZOffset=0  TranslationZOffsetUnits=m  TranslationThetaOffset=0  TranslationThetaOffsetUnits=deg  RotationMethod=StandardAxis  RotationAngleUnits=deg  RotationStandardAxis=-X  RotationAngle=90  RotationArbitraryAxis=[0 0 1]  FollAlignAxisA=+X  BaseAlignAxisA=+Y  FollAlignAxisB=+Y  BaseAlignAxisB=+Z  RotationSequenceAxes=FollowerAxes  RotationSequence=XYX  RotationSequenceAngles=[0 0 0]  RotationSequenceAnglesUnits=deg  RotationMatrix=[1 0 0; 0 1 0; 0 0 1]
  Rigid Transform2 : sm_lib/Frames and Transforms/Rigid Transform  TranslationMethod=Cartesian  TranslationStandardOffset=L/2  TranslationLengthUnit=cm  TranslationStandardAxis=-X  TranslationCartesianOffset=[L/2-Lo -W/2 -H/2+Lh]  TranslationROffset=0  TranslationROffsetUnits=m  TranslationZOffset=0  TranslationZOffsetUnits=m  TranslationThetaOffset=0  TranslationThetaOffsetUnits=deg  RotationMethod=StandardAxis  RotationAngleUnits=deg  RotationStandardAxis=-X  RotationAngle=90  RotationArbitraryAxis=[0 0 1]  FollAlignAxisA=+X  BaseAlignAxisA=+Y  FollAlignAxisB=+Y  BaseAlignAxisB=+Z  RotationSequenceAxes=FollowerAxes  RotationSequence=XYX  RotationSequenceAngles=[0 0 0]  RotationSequenceAnglesUnits=deg  RotationMatrix=[1 0 0; 0 1 0; 0 0 1]
  Rigid Transform3 : sm_lib/Frames and Transforms/Rigid Transform  TranslationMethod=Cartesian  TranslationStandardOffset=L/2  TranslationLengthUnit=cm  TranslationStandardAxis=-X  TranslationCartesianOffset=[-L/2+Lo -W/2 -H/2+Lh]  TranslationROffset=0  TranslationROffsetUnits=m  TranslationZOffset=0  TranslationZOffsetUnits=m  TranslationThetaOffset=0  TranslationThetaOffsetUnits=deg  RotationMethod=StandardAxis  RotationAngleUnits=deg  RotationStandardAxis=-X  RotationAngle=90  RotationArbitraryAxis=[0 0 1]  FollAlignAxisA=+X  BaseAlignAxisA=+Y  FollAlignAxisB=+Y  BaseAlignAxisB=+Z  RotationSequenceAxes=FollowerAxes  RotationSequence=XYX  RotationSequenceAngles=[0 0 0]  RotationSequenceAnglesUnits=deg  RotationMatrix=[1 0 0; 0 1 0; 0 0 1]
  Rigid Transform4 : sm_lib/Frames and Transforms/Rigid Transform  TranslationMethod=Cartesian  TranslationStandardOffset=L/2  TranslationLengthUnit=cm  TranslationStandardAxis=-X  TranslationCartesianOffset=[L/2 -W/2 -H/2]  TranslationROffset=0  TranslationROffsetUnits=m  TranslationZOffset=0  TranslationZOffsetUnits=m  TranslationThetaOffset=0  TranslationThetaOffsetUnits=deg  RotationMethod=StandardAxis  RotationAngleUnits=deg  RotationStandardAxis=-X  RotationAngle=90  RotationArbitraryAxis=[0 0 1]  FollAlignAxisA=+X  BaseAlignAxisA=+Y  FollAlignAxisB=+Y  BaseAlignAxisB=+Z  RotationSequenceAxes=FollowerAxes  RotationSequence=XYX  RotationSequenceAngles=[0 0 0]  RotationSequenceAnglesUnits=deg  RotationMatrix=[1 0 0; 0 1 0; 0 0 1]
  Rigid Transform5 : sm_lib/Frames and Transforms/Rigid Transform  TranslationMethod=Cartesian  TranslationStandardOffset=L/2  TranslationLengthUnit=cm  TranslationStandardAxis=-X  TranslationCartesianOffset=[-L/2 -W/2 -H/2]  TranslationROffset=0  TranslationROffsetUnits=m  TranslationZOffset=0  TranslationZOffsetUnits=m  TranslationThetaOffset=0  TranslationThetaOffsetUnits=deg  RotationMethod=StandardAxis  RotationAngleUnits=deg  RotationStandardAxis=-X  RotationAngle=90  RotationArbitraryAxis=[0 0 1]  FollAlignAxisA=+X  BaseAlignAxisA=+Y  FollAlignAxisB=+Y  BaseAlignAxisB=+Z  RotationSequenceAxes=FollowerAxes  RotationSequence=XYX  RotationSequenceAngles=[0 0 0]  RotationSequenceAnglesUnits=deg  RotationMatrix=[1 0 0; 0 1 0; 0 0 1]
  Rigid Transform6 : sm_lib/Frames and Transforms/Rigid Transform  TranslationMethod=Cartesian  TranslationStandardOffset=L/2  TranslationLengthUnit=cm  TranslationStandardAxis=-X  TranslationCartesianOffset=[L/2 W/2 -H/2]  TranslationROffset=0  TranslationROffsetUnits=m  TranslationZOffset=0  TranslationZOffsetUnits=m  TranslationThetaOffset=0  TranslationThetaOffsetUnits=deg  RotationMethod=StandardAxis  RotationAngleUnits=deg  RotationStandardAxis=-X  RotationAngle=90  RotationArbitraryAxis=[0 0 1]  FollAlignAxisA=+X  BaseAlignAxisA=+Y  FollAlignAxisB=+Y  BaseAlignAxisB=+Z  RotationSequenceAxes=FollowerAxes  RotationSequence=XYX  RotationSequenceAngles=[0 0 0]  RotationSequenceAnglesUnits=deg  RotationMatrix=[1 0 0; 0 1 0; 0 0 1]
  Rigid Transform7 : sm_lib/Frames and Transforms/Rigid Transform  TranslationMethod=Cartesian  TranslationStandardOffset=L/2  TranslationLengthUnit=cm  TranslationStandardAxis=+X  TranslationCartesianOffset=[-L/2 W/2 -H/2]  TranslationROffset=0  TranslationROffsetUnits=m  TranslationZOffset=0  TranslationZOffsetUnits=m  TranslationThetaOffset=0  TranslationThetaOffsetUnits=deg  RotationMethod=StandardAxis  RotationAngleUnits=deg  RotationStandardAxis=-X  RotationAngle=90  RotationArbitraryAxis=[0 0 1]  FollAlignAxisA=+X  BaseAlignAxisA=+Y  FollAlignAxisB=+Y  BaseAlignAxisB=+Z  RotationSequenceAxes=FollowerAxes  RotationSequence=XYX  RotationSequenceAngles=[0 0 0]  RotationSequenceAnglesUnits=deg  RotationMatrix=[1 0 0; 0 1 0; 0 0 1]
  Rigid Transform8 : sm_lib/Frames and Transforms/Rigid Transform  TranslationMethod=Cartesian  TranslationStandardOffset=L/2  TranslationLengthUnit=cm  TranslationStandardAxis=-X  TranslationCartesianOffset=[L/2 -W/2 H/2]  TranslationROffset=0  TranslationROffsetUnits=m  TranslationZOffset=0  TranslationZOffsetUnits=m  TranslationThetaOffset=0  TranslationThetaOffsetUnits=deg  RotationMethod=StandardAxis  RotationAngleUnits=deg  RotationStandardAxis=-X  RotationAngle=90  RotationArbitraryAxis=[0 0 1]  FollAlignAxisA=+X  BaseAlignAxisA=+Y  FollAlignAxisB=+Y  BaseAlignAxisB=+Z  RotationSequenceAxes=FollowerAxes  RotationSequence=XYX  RotationSequenceAngles=[0 0 0]  RotationSequenceAnglesUnits=deg  RotationMatrix=[1 0 0; 0 1 0; 0 0 1]
  Rigid Transform9 : sm_lib/Frames and Transforms/Rigid Transform  TranslationMethod=Cartesian  TranslationStandardOffset=L/2  TranslationLengthUnit=cm  TranslationStandardAxis=-X  TranslationCartesianOffset=[-L/2 -W/2 H/2]  TranslationROffset=0  TranslationROffsetUnits=m  TranslationZOffset=0  TranslationZOffsetUnits=m  TranslationThetaOffset=0  TranslationThetaOffsetUnits=deg  RotationMethod=StandardAxis  RotationAngleUnits=deg  RotationStandardAxis=-X  RotationAngle=90  RotationArbitraryAxis=[0 0 1]  FollAlignAxisA=+X  BaseAlignAxisA=+Y  FollAlignAxisB=+Y  BaseAlignAxisB=+Z  RotationSequenceAxes=FollowerAxes  RotationSequence=XYX  RotationSequenceAngles=[0 0 0]  RotationSequenceAnglesUnits=deg  RotationMatrix=[1 0 0; 0 1 0; 0 0 1]
  Solver Configuration : nesl_utility/Solver Configuration  PhysicalDomain=network_engine_domain  SubClassName=solver  LeftPortType=input  RightPortType=generic  Tones=[]  Harmonics=[]  SimulateNoise=off  Profile=off  UseLocalSampling=off  EnableSwitchedLinearOptims=on  FrequencyDomain=off  UseCCode=off  RelTol=0.001  AbsTol=1e-06  MinStep=1e-09  ToWorkspace=off  RevertToSquareIcSolve=off  NumHomotopyIterations=100  PhasorMode=off  PhasorModeNumHarmonics=1  DoDC=off  ResidualTolerance=1e-09  UseLocalSolver=off  LocalSolverChoice=NE_BACKWARD_EULER_ADVANCER  LocalSolverSampleTime=0.001  DoFixedCost=off  MaxNonlinIter=3  MaxModeIter=2  ComputeImpulses=off  ImpulseIterations=2  LinearAlgebra=Sparse  EquationFormulation=NE_TIME_EF  DelaysMemoryBudget=1024  AutomaticFiltering=on  FilteringTimeConstant=0.001  PartitionStorageMethod=AS_NEEDED  PartitionMemoryBudget=1024  PartitionMethod=FAST
  Spatial Contact Force{,1..7} (8 alike) : sm_lib/Forces and Torques/Spatial Contact Force  CoefficientOfDynamicFriction=0.3  CoefficientOfStaticFriction=0.5  NormalDamping=1e3  NormalDampingUnits=N/(m/s)  NormalStiffness=1e6  NormalStiffnessUnits=N/m  FrictionalCriticalVelocity=1e-3  FrictionalCriticalVelocityUnits=m/s  ZeroCrossDetectContactStartAndEnd=off  SenseFrictionalForceMagnitude=off  SenseNormalForceMagnitude=off  SenseSeparationDistance=off  NormalTransitionRegionWidth=1e-4  NormalTransitionRegionWidthUnits=m  FrictionType=SmoothStickSlip
  Spherical Solid{,1..7} (8 alike) : sm_lib/Body Elements/Spherical Solid  GraphicAmbientColor=[0.15 0.15 0.15 1.0]  BasedOnType=Density  CenterOfMass=[0 0 0]  CenterOfMassUnits=m  GraphicDiffuseColor=[0.5 0.5 0.5]  Density=1000  DensityUnits=kg/m^3  DoExposeReferenceFrame=on  GraphicEmissiveColor=[0.0 0.0 0.0 1.0]  ExportEntireGeometry=on  SerializedExposedGeometries=<ExposedGeometries><ExposedGeometry><RawGeometryId>entire</RawGeometryId><ExposedGeometryId>G</ExposedGeometryId></ExposedGeometry></ExposedGeometries>  SerializedFrames=<Frames/>  MarkerShape=Sphere  MarkerSize=10  GraphicType=FromGeometry  InertiaType=CalculateFromGeometry  Mass=1  MassUnits=kg  MomentsOfInertia=[1 1 1]  MomentsOfInertiaUnits=kg*m^2  GraphicOpacity=1.0  ProductsOfInertia=[0 0 0]  ProductsOfInertiaUnits=kg*m^2  GraphicShininess=75  GraphicSpecularColor=[0.5 0.5 0.5 1.0]  SphereRadius=0.1  SphereRadiusUnits=cm  GraphicVisPropType=SimpleVisualProperties
  To Workspace : ToWorkspace  VariableName=axis  SaveFormat=Timeseries  SampleTime=1
      settings: MaxDataPoints=200
  To Workspace1 : ToWorkspace  VariableName=q  SaveFormat=Timeseries  SampleTime=1
      settings: MaxDataPoints=200
  To Workspace2 : ToWorkspace  VariableName=distance_forward  SaveFormat=Timeseries  SampleTime=1
      settings: MaxDataPoints=200
  Torso : sm_lib/Body Elements/Brick Solid  GraphicAmbientColor=[0.15 0.15 0.15 1.0]  BasedOnType=Mass  BrickDimensions=[L W H]  BrickDimensionUnits=cm  CenterOfMass=[0 0 0]  CenterOfMassUnits=m  GraphicDiffuseColor=rgb  Density=1000  DensityUnits=kg/m^3  DoExposeReferenceFrame=on  GraphicEmissiveColor=[0.0 0.0 0.0 1.0]  ExportEntireGeometry=off  SerializedFrames=<Frames/>  MarkerShape=Sphere  MarkerSize=10  GraphicType=FromGeometry  InertiaType=CalculateFromGeometry  Mass=weight  MassUnits=kg  MomentsOfInertia=[1 1 1]  MomentsOfInertiaUnits=kg*m^2  GraphicOpacity=1.0  ProductsOfInertia=[0 0 0]  ProductsOfInertiaUnits=kg*m^2  GraphicShininess=75  GraphicSpecularColor=[0.5 0.5 0.5 1.0]  GraphicVisPropType=SimpleVisualProperties
  Transform Sensor : sm_lib/Frames and Transforms/Transform Sensor  MeasurementFrame=World  SenseAngle=on  SenseAxis=on  SenseAngle1=off  SenseAngle2=off  SenseAngle3=off  SenseQ=off  SenseR=off  SenseOmegaX=off  SenseOmegaY=off  SenseOmegaZ=off  SenseOmega1=off  SenseOmega2=off  SenseOmega3=off  SenseQDot=off  SenseRDot=off  SenseAlphaX=off  SenseAlphaY=off  SenseAlphaZ=off  SenseAlpha1=off  SenseAlpha2=off  SenseAlpha3=off  SenseQDDot=off  SenseRDDot=off  SenseX=on  SenseY=off  SenseZ=off  SenseRad=off  SenseAzim=off  SenseDist=off  SenseInc=off  SenseXDot=off  SenseYDot=off  SenseZDot=off  SenseRadDot=off  SenseAzimDot=off  SenseDistDot=off  SenseIncDot=off  SenseXDDot=off  SenseYDDot=off  SenseZDDot=off  SenseRadDDot=off  SenseAzimDDot=off  SenseDistDDot=off  SenseIncDDot=off
  World Frame1 : sm_lib/Frames and Transforms/World Frame
  World Frame : PMIOPort  Side=Left
  Front Right Leg : PMIOPort  Port=2  Side=Right
  Front Left Leg : PMIOPort  Port=3  Side=Right
  Back Right Leg : PMIOPort  Port=4  Side=Right
  Back Left Leg : PMIOPort  Port=5  Side=Right
  Ground : PMIOPort  Port=6  Side=Left
  wires:
  PS-Simulink Converter/1 -> To Workspace/1
  PS-Simulink Converter1/1 -> To Workspace1/1
  PS-Simulink Converter2/1 -> To Workspace2/1
  connections:
  Rigid Transform/RConn1 -- Back Right Leg/RConn1
  Rigid Transform1/RConn1 -- Front Right Leg/RConn1
  Back Left Leg/RConn1 -- Rigid Transform3/RConn1
  Front Left Leg/RConn1 -- Rigid Transform2/RConn1
  Spherical Solid2/RConn1 -- Rigid Transform6/RConn1
  Rigid Transform7/RConn1 -- Spherical Solid3/RConn1
  Rigid Transform4/RConn1 -- Spherical Solid/RConn1
  Spherical Solid1/RConn1 -- Rigid Transform5/RConn1
  Spherical Solid/LConn1 -- Spatial Contact Force1/LConn1
  Spherical Solid1/LConn1 -- Spatial Contact Force/LConn1
  Spatial Contact Force2/LConn1 -- Spherical Solid2/LConn1
  Spatial Contact Force3/LConn1 -- Spherical Solid3/LConn1
  Spatial Contact Force/RConn1 -- Spatial Contact Force4/RConn1 -- Spatial Contact Force5/RConn1 -- Spatial Contact Force1/RConn1 -- Spatial Contact Force7/RConn1 -- Spatial Contact Force6/RConn1 -- Spatial Contact Force2/RConn1 -- Spatial Contact Force3/RConn1 -- Ground/RConn1
  Spatial Contact Force7/LConn1 -- Spherical Solid7/LConn1
  Rigid Transform11/RConn1 -- Spherical Solid7/RConn1
  Spherical Solid4/LConn1 -- Spatial Contact Force5/LConn1
  Spherical Solid6/RConn1 -- Rigid Transform10/RConn1
  Spherical Solid5/LConn1 -- Spatial Contact Force4/LConn1
  Rigid Transform8/RConn1 -- Spherical Solid4/RConn1
  Spherical Solid5/RConn1 -- Rigid Transform9/RConn1
  Spatial Contact Force6/LConn1 -- Spherical Solid6/LConn1
  Rigid Transform1/LConn1 -- 6-DOF Joint/RConn1 -- Transform Sensor/RConn1 -- Torso/RConn1 -- Solver Configuration/RConn1 -- Mechanism Configuration/RConn1 -- Rigid Transform2/LConn1 -- Rigid Transform7/LConn1 -- Rigid Transform5/LConn1 -- Rigid Transform6/LConn1 -- Rigid Transform4/LConn1 -- Rigid Transform11/LConn1 -- Rigid Transform9/LConn1 -- Rigid Transform8/LConn1 -- Rigid Transform10/LConn1 -- Rigid Transform/LConn1 -- Rigid Transform3/LConn1
  6-DOF Joint/LConn1 -- World Frame/RConn1
  Transform Sensor/LConn1 -- World Frame1/RConn1
  Transform Sensor/RConn4 -- PS-Simulink Converter2/LConn1
  Transform Sensor/RConn3 -- PS-Simulink Converter/LConn1
  Transform Sensor/RConn2 -- PS-Simulink Converter1/LConn1
